simulink subsystem "Pack_SOC_Estimation"  (R2021a)
settings: Solver=VariableStepAuto  StartTime=0.0  StopTime=10.0  RelTol=1e-3
(part 1 of 4)
settings Model: Creator=mirko  LastModifiedBy=mirko

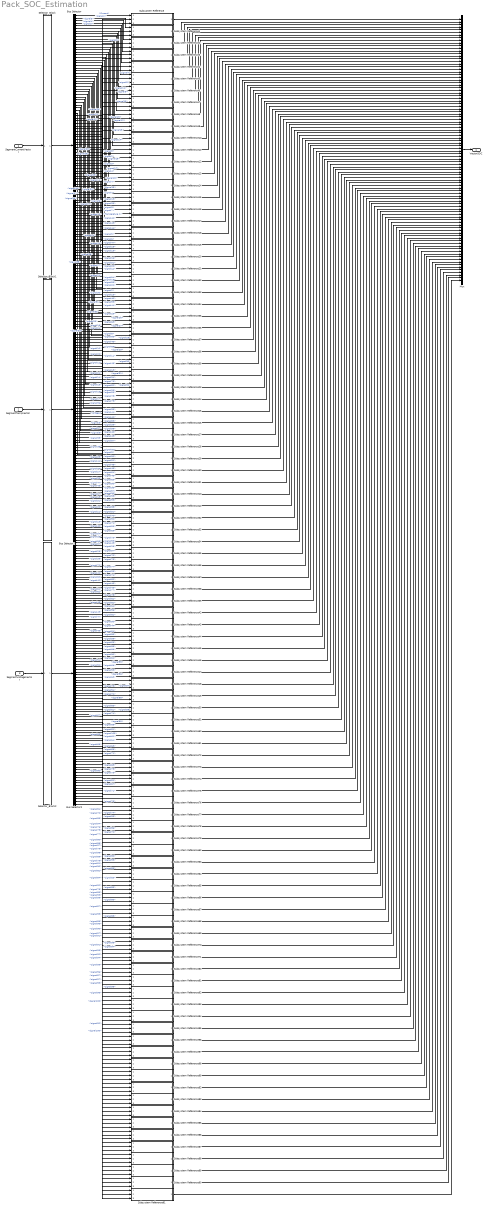
== system Pack_SOC_Estimation ==
  SegmentCurrentVector : Inport
  SegmentTempVector : Inport  Port=2
  SegmentVoltageVector : Inport  Port=3
  Bus Selector : BusSelector  OutputSignals=Current,signal2,signal3,signal4,signal5,signal6,signal7,signal8,signal9,signal10,signal11,signal12,signal13,signal14,signal15,signal16,signal17,signal18,signal19,signal20,signal21,signal22,signal23,signal24,signal25,signal26,signal27,signal28,signal29,signal30,signal31,signal32,signal33,signal34,signal35,signal36,signal37,signal38,signal39,signal40,signal41,signal42,signal43,signal44,signal45,signal46,signal47,signal48,signal49,signal50,signal51,signal52,signal53,signal54,signal55,signal56,signal57,signal58,signal59,signal60,signal61,signal62,signal63,signal64,signal65,signal66,signal67,signal68,signal69,signal70,signal71,signal72,signal73,signal74,signal75,signal76,signal77,signal78,signal79,signal80,signal81,signal82,signal83,signal84,signal85,signal86,signal87,signal88,signal89,signal90,signal91,signal92,signal93,signal94,signal95,signal96,signal97,signal98,signal99,signal100
  Bus Selector1 : BusSelector  OutputSignals=Temperature K,signal2,signal3,signal4,signal5,signal6,signal7,signal8,signal9,signal10,signal11,signal12,signal13,signal14,signal15,signal16,signal17,signal18,signal19,signal20,signal21,signal22,signal23,signal24,signal25,signal26,signal27,signal28,signal29,signal30,signal31,signal32,signal33,signal34,signal35,signal36,signal37,signal38,signal39,signal40,signal41,signal42,signal43,signal44,signal45,signal46,signal47,signal48,signal49,signal50,signal51,signal52,signal53,signal54,signal55,signal56,signal57,signal58,signal59,signal60,signal61,signal62,signal63,signal64,signal65,signal66,signal67,signal68,signal69,signal70,signal71,signal72,signal73,signal74,signal75,signal76,signal77,signal78,signal79,signal80,signal81,signal82,signal83,signal84,signal85,signal86,signal87,signal88,signal89,signal90,signal91,signal92,signal93,signal94,signal95,signal96,signal97,signal98,signal99,signal100
  Bus Selector2 : BusSelector  OutputSignals=Voltage,signal2,signal3,signal4,signal5,signal6,signal7,signal8,signal9,signal10,signal11,signal12,signal13,signal14,signal15,signal16,signal17,signal18,signal19,signal20,signal21,signal22,signal23,signal24,signal25,signal26,signal27,signal28,signal29,signal30,signal31,signal32,signal33,signal34,signal35,signal36,signal37,signal38,signal39,signal40,signal41,signal42,signal43,signal44,signal45,signal46,signal47,signal48,signal49,signal50,signal51,signal52,signal53,signal54,signal55,signal56,signal57,signal58,signal59,signal60,signal61,signal62,signal63,signal64,signal65,signal66,signal67,signal68,signal69,signal70,signal71,signal72,signal73,signal74,signal75,signal76,signal77,signal78,signal79,signal80,signal81,signal82,signal83,signal84,signal85,signal86,signal87,signal88,signal89,signal90,signal91,signal92,signal93,signal94,signal95,signal96,signal97,signal98,signal99,signal100
  Mux : Mux  Inputs=100
  Selector_Block : Subsystem
  Selector_Block1 : Subsystem
  Selector_Block2 : Subsystem
  Subsystem Reference{,1..99} (100 alike) : Subsystem  ReferencedSubsystem=Single_Cell_SOC_Estimation
  VectorSOC : Outport
  wires:
  SegmentCurrentVector/1 -> Selector_Block/1(In1)
  SegmentTempVector/1 -> Selector_Block1/1(In1)
  SegmentVoltageVector/1 -> Selector_Block2/1(In1)
  Bus Selector/1 -> Subsystem Reference/1  "<Current>"
  Bus Selector/2 -> Subsystem Reference1/1  "<signal2>"
  Bus Selector/3 -> Subsystem Reference2/1  "<signal3>"
  Bus Selector/4 -> Subsystem Reference3/1  "<signal4>"
  Bus Selector/5 -> Subsystem Reference4/1  "<signal5>"
  Bus Selector/6 -> Subsystem Reference5/1  "<signal6>"
  Bus Selector/7 -> Subsystem Reference6/1  "<signal7>"
  Bus Selector/8 -> Subsystem Reference7/1  "<signal8>"
  Bus Selector/9 -> Subsystem Reference8/1  "<signal9>"
  Bus Selector/10 -> Subsystem Reference9/1  "<signal10>"
  Bus Selector/11 -> Subsystem Reference10/1  "<signal11>"
  Bus Selector/12 -> Subsystem Reference11/1  "<signal12>"
  Bus Selector/13 -> Subsystem Reference12/1  "<signal13>"
  Bus Selector/14 -> Subsystem Reference13/1  "<signal14>"
  Bus Selector/15 -> Subsystem Reference14/1  "<signal15>"
  Bus Selector/16 -> Subsystem Reference15/1  "<signal16>"
  Bus Selector/17 -> Subsystem Reference16/1  "<signal17>"
  Bus Selector/18 -> Subsystem Reference17/1  "<signal18>"
  Bus Selector/19 -> Subsystem Reference18/1  "<signal19>"
  Bus Selector/20 -> Subsystem Reference19/1  "<signal20>"
  Bus Selector/21 -> Subsystem Reference20/1  "<signal21>"
  Bus Selector/22 -> Subsystem Reference21/1  "<signal22>"
  Bus Selector/23 -> Subsystem Reference32/1  "<signal23>"
  Bus Selector/24 -> Subsystem Reference33/1  "<signal24>"
  Bus Selector/25 -> Subsystem Reference34/1  "<signal25>"
  Bus Selector/26 -> Subsystem Reference35/1  "<signal26>"
  Bus Selector/27 -> Subsystem Reference36/1  "<signal27>"
  Bus Selector/28 -> Subsystem Reference37/1  "<signal28>"
  Bus Selector/29 -> Subsystem Reference38/1  "<signal29>"
  Bus Selector/30 -> Subsystem Reference39/1  "<signal30>"
  Bus Selector/31 -> Subsystem Reference22/1  "<signal31>"
  Bus Selector/32 -> Subsystem Reference23/1  "<signal32>"
  Bus Selector/33 -> Subsystem Reference24/1  "<signal33>"
  Bus Selector/34 -> Subsystem Reference25/1  "<signal34>"
  Bus Selector/35 -> Subsystem Reference26/1  "<signal35>"
  Bus Selector/36 -> Subsystem Reference27/1  "<signal36>"
  Bus Selector/37 -> Subsystem Reference28/1  "<signal37>"
  Bus Selector/38 -> Subsystem Reference29/1  "<signal38>"
  Bus Selector/39 -> Subsystem Reference30/1  "<signal39>"
  Bus Selector/40 -> Subsystem Reference31/1  "<signal40>"
  Bus Selector/41 -> Subsystem Reference40/1  "<signal41>"
  Bus Selector/42 -> Subsystem Reference41/1  "<signal42>"
  Bus Selector/43 -> Subsystem Reference52/1  "<signal43>"
  Bus Selector/44 -> Subsystem Reference53/1  "<signal44>"
  Bus Selector/45 -> Subsystem Reference54/1  "<signal45>"
  Bus Selector/46 -> Subsystem Reference55/1  "<signal46>"
  Bus Selector/47 -> Subsystem Reference56/1  "<signal47>"
  Bus Selector/48 -> Subsystem Reference57/1  "<signal48>"
  Bus Selector/49 -> Subsystem Reference58/1  "<signal49>"
  Bus Selector/50 -> Subsystem Reference59/1  "<signal50>"
  Bus Selector/65 -> Subsystem Reference74/1  "<signal65>"
  Bus Selector/87 -> Subsystem Reference96/1  "<signal87>"
  Bus Selector/97 -> Subsystem Reference88/1  "<signal97>"
  Bus Selector/89 -> Subsystem Reference98/1  "<signal89>"
  Bus Selector/81 -> Subsystem Reference80/1  "<signal81>"
  Bus Selector/90 -> Subsystem Reference99/1  "<signal90>"
  Bus Selector/59 -> Subsystem Reference50/1  "<signal59>"
  Bus Selector/78 -> Subsystem Reference69/1  "<signal78>"
  Bus Selector/86 -> Subsystem Reference95/1  "<signal86>"
  Bus Selector/93 -> Subsystem Reference84/1  "<signal93>"
  Bus Selector/92 -> Subsystem Reference83/1  "<signal92>"
  Bus Selector/52 -> Subsystem Reference43/1  "<signal52>"
  Bus Selector/88 -> Subsystem Reference97/1  "<signal88>"
  Bus Selector/51 -> Subsystem Reference42/1  "<signal51>"
  Bus Selector/54 -> Subsystem Reference45/1  "<signal54>"
  Bus Selector/98 -> Subsystem Reference89/1  "<signal98>"
  Bus Selector/80 -> Subsystem Reference71/1  "<signal80>"
  Bus Selector/84 -> Subsystem Reference93/1  "<signal84>"
  Bus Selector/62 -> Subsystem Reference61/1  "<signal62>"
  Bus Selector/70 -> Subsystem Reference79/1  "<signal70>"
  Bus Selector/83 -> Subsystem Reference92/1  "<signal83>"
  Bus Selector/75 -> Subsystem Reference66/1  "<signal75>"
  Bus Selector/76 -> Subsystem Reference67/1  "<signal76>"
  Bus Selector/68 -> Subsystem Reference77/1  "<signal68>"
  Bus Selector/66 -> Subsystem Reference75/1  "<signal66>"
  Bus Selector/82 -> Subsystem Reference81/1  "<signal82>"
  Bus Selector/69 -> Subsystem Reference78/1  "<signal69>"
  Bus Selector/73 -> Subsystem Reference64/1  "<signal73>"
  Bus Selector/56 -> Subsystem Reference47/1  "<signal56>"
  Bus Selector/96 -> Subsystem Reference87/1  "<signal96>"
  Bus Selector/55 -> Subsystem Reference46/1  "<signal55>"
  Bus Selector/60 -> Subsystem Reference51/1  "<signal60>"
  Bus Selector/95 -> Subsystem Reference86/1  "<signal95>"
  Bus Selector/61 -> Subsystem Reference60/1  "<signal61>"
  Bus Selector/64 -> Subsystem Reference73/1  "<signal64>"
  Bus Selector/99 -> Subsystem Reference90/1  "<signal99>"
  Bus Selector/85 -> Subsystem Reference94/1  "<signal85>"
  Bus Selector/100 -> Subsystem Reference91/1  "<signal100>"
  Bus Selector/79 -> Subsystem Reference70/1  "<signal79>"
  Bus Selector/72 -> Subsystem Reference63/1  "<signal72>"
  Bus Selector/77 -> Subsystem Reference68/1  "<signal77>"
  Bus Selector/63 -> Subsystem Reference72/1  "<signal63>"
  Bus Selector/74 -> Subsystem Reference65/1  "<signal74>"
  Bus Selector/57 -> Subsystem Reference48/1  "<signal57>"
  Bus Selector/71 -> Subsystem Reference62/1  "<signal71>"
  Bus Selector/53 -> Subsystem Reference44/1  "<signal53>"
  Bus Selector/58 -> Subsystem Reference49/1  "<signal58>"
  Bus Selector/94 -> Subsystem Reference85/1  "<signal94>"
  Bus Selector/67 -> Subsystem Reference76/1  "<signal67>"
  Bus Selector/91 -> Subsystem Reference82/1  "<signal91>"
  Bus Selector1/79 -> Subsystem Reference70/2  "<signal79>"
  Bus Selector1/69 -> Subsystem Reference78/2  "<signal69>"
  Bus Selector1/67 -> Subsystem Reference76/2  "<signal67>"
  Bus Selector1/66 -> Subsystem Reference75/2  "<signal66>"
  Bus Selector1/46 -> Subsystem Reference55/2  "<signal46>"
  Bus Selector1/70 -> Subsystem Reference79/2  "<signal70>"
  Bus Selector1/24 -> Subsystem Reference33/2  "<signal24>"
  Bus Selector1/29 -> Subsystem Reference38/2  "<signal29>"
  Bus Selector1/37 -> Subsystem Reference28/2  "<signal37>"
  Bus Selector1/47 -> Subsystem Reference56/2  "<signal47>"
  Bus Selector1/39 -> Subsystem Reference30/2  "<signal39>"
  Bus Selector1/31 -> Subsystem Reference22/2  "<signal31>"
  Bus Selector1/40 -> Subsystem Reference31/2  "<signal40>"
  Bus Selector1/27 -> Subsystem Reference36/2  "<signal27>"
  Bus Selector1/23 -> Subsystem Reference32/2  "<signal23>"
  Bus Selector1/9 -> Subsystem Reference8/2  "<signal9>"
  Bus Selector1/75 -> Subsystem Reference66/2  "<signal75>"
  Bus Selector1/78 -> Subsystem Reference69/2  "<signal78>"
  Bus Selector1/77 -> Subsystem Reference68/2  "<signal77>"
  Bus Selector1/25 -> Subsystem Reference34/2  "<signal25>"
  Bus Selector1/76 -> Subsystem Reference67/2  "<signal76>"
  Bus Selector1/61 -> Subsystem Reference60/2  "<signal61>"
  Bus Selector1/62 -> Subsystem Reference61/2  "<signal62>"
  Bus Selector1/65 -> Subsystem Reference74/2  "<signal65>"
  Bus Selector1/63 -> Subsystem Reference72/2  "<signal63>"
  Bus Selector1/80 -> Subsystem Reference71/2  "<signal80>"
  Bus Selector1/53 -> Subsystem Reference44/2  "<signal53>"
  Bus Selector1/52 -> Subsystem Reference43/2  "<signal52>"
  Bus Selector1/51 -> Subsystem Reference42/2  "<signal51>"
  Bus Selector1/54 -> Subsystem Reference45/2  "<signal54>"
  Bus Selector1/93 -> Subsystem Reference84/2  "<signal93>"
  Bus Selector1/94 -> Subsystem Reference85/2  "<signal94>"
  Bus Selector1/91 -> Subsystem Reference82/2  "<signal91>"
  Bus Selector1/82 -> Subsystem Reference81/2  "<signal82>"
  Bus Selector1/81 -> Subsystem Reference80/2  "<signal81>"
  Bus Selector1/28 -> Subsystem Reference37/2  "<signal28>"
  Bus Selector1/57 -> Subsystem Reference48/2  "<signal57>"
  Bus Selector1/72 -> Subsystem Reference63/2  "<signal72>"
  Bus Selector1/96 -> Subsystem Reference87/2  "<signal96>"
  Bus Selector1/36 -> Subsystem Reference27/2  "<signal36>"
  Bus Selector1/90 -> Subsystem Reference99/2  "<signal90>"
  Bus Selector1/83 -> Subsystem Reference92/2  "<signal83>"
  Bus Selector1/71 -> Subsystem Reference62/2  "<signal71>"
  Bus Selector1/15 -> Subsystem Reference14/2  "<signal15>"
  Bus Selector1/100 -> Subsystem Reference91/2  "<signal100>"
  Bus Selector1/73 -> Subsystem Reference64/2  "<signal73>"
  Bus Selector1/99 -> Subsystem Reference90/2  "<signal99>"
  Bus Selector1/98 -> Subsystem Reference89/2  "<signal98>"
  Bus Selector1/43 -> Subsystem Reference52/2  "<signal43>"
  Bus Selector1/56 -> Subsystem Reference47/2  "<signal56>"
  Bus Selector1/42 -> Subsystem Reference41/2  "<signal42>"
  Bus Selector1/2 -> Subsystem Reference1/2  "<signal2>"
  Bus Selector1/38 -> Subsystem Reference29/2  "<signal38>"
  Bus Selector1/95 -> Subsystem Reference86/2  "<signal95>"
  Bus Selector1/59 -> Subsystem Reference50/2  "<signal59>"
  Bus Selector1/1 -> Subsystem Reference/2  "<Temperature K>"
  Bus Selector1/58 -> Subsystem Reference49/2  "<signal58>"
  Bus Selector1/4 -> Subsystem Reference3/2  "<signal4>"
  Bus Selector1/88 -> Subsystem Reference97/2  "<signal88>"
  Bus Selector1/48 -> Subsystem Reference57/2  "<signal48>"
  Bus Selector1/30 -> Subsystem Reference39/2  "<signal30>"
  Bus Selector1/34 -> Subsystem Reference25/2  "<signal34>"
  Bus Selector1/84 -> Subsystem Reference93/2  "<signal84>"
  Bus Selector1/86 -> Subsystem Reference95/2  "<signal86>"
  Bus Selector1/12 -> Subsystem Reference11/2  "<signal12>"
  Bus Selector1/20 -> Subsystem Reference19/2  "<signal20>"
  Bus Selector1/33 -> Subsystem Reference24/2  "<signal33>"
  Bus Selector1/26 -> Subsystem Reference35/2  "<signal26>"
  Bus Selector1/89 -> Subsystem Reference98/2  "<signal89>"
  Bus Selector1/18 -> Subsystem Reference17/2  "<signal18>"
  Bus Selector1/16 -> Subsystem Reference15/2  "<signal16>"
  Bus Selector1/85 -> Subsystem Reference94/2  "<signal85>"
  Bus Selector1/74 -> Subsystem Reference65/2  "<signal74>"
  Bus Selector1/32 -> Subsystem Reference23/2  "<signal32>"
  Bus Selector1/68 -> Subsystem Reference77/2  "<signal68>"
  Bus Selector1/97 -> Subsystem Reference88/2  "<signal97>"
  Bus Selector1/19 -> Subsystem Reference18/2  "<signal19>"
  Bus Selector1/6 -> Subsystem Reference5/2  "<signal6>"
  Bus Selector1/5 -> Subsystem Reference4/2  "<signal5>"
  Bus Selector1/10 -> Subsystem Reference9/2  "<signal10>"
  Bus Selector1/45 -> Subsystem Reference54/2  "<signal45>"
  Bus Selector1/11 -> Subsystem Reference10/2  "<signal11>"
  Bus Selector1/14 -> Subsystem Reference13/2  "<signal14>"
  Bus Selector1/49 -> Subsystem Reference58/2  "<signal49>"
  Bus Selector1/60 -> Subsystem Reference51/2  "<signal60>"
  Bus Selector1/35 -> Subsystem Reference26/2  "<signal35>"
  Bus Selector1/64 -> Subsystem Reference73/2  "<signal64>"
  Bus Selector1/50 -> Subsystem Reference59/2  "<signal50>"
  Bus Selector1/22 -> Subsystem Reference21/2  "<signal22>"
  Bus Selector1/13 -> Subsystem Reference12/2  "<signal13>"
  Bus Selector1/7 -> Subsystem Reference6/2  "<signal7>"
  Bus Selector1/21 -> Subsystem Reference20/2  "<signal21>"
  Bus Selector1/3 -> Subsystem Reference2/2  "<signal3>"
  Bus Selector1/8 -> Subsystem Reference7/2  "<signal8>"
  Bus Selector1/55 -> Subsystem Reference46/2  "<signal55>"
  Bus Selector1/44 -> Subsystem Reference53/2  "<signal44>"
  Bus Selector1/92 -> Subsystem Reference83/2  "<signal92>"
  Bus Selector1/17 -> Subsystem Reference16/2  "<signal17>"
  Bus Selector1/41 -> Subsystem Reference40/2  "<signal41>"
  Bus Selector1/87 -> Subsystem Reference96/2  "<signal87>"
  Bus Selector2/79 -> Subsystem Reference70/3  "<signal79>"
  Bus Selector2/69 -> Subsystem Reference78/3  "<signal69>"
  Bus Selector2/67 -> Subsystem Reference76/3  "<signal67>"
  Bus Selector2/66 -> Subsystem Reference75/3  "<signal66>"
  Bus Selector2/46 -> Subsystem Reference55/3  "<signal46>"
  Bus Selector2/70 -> Subsystem Reference79/3  "<signal70>"
  Bus Selector2/24 -> Subsystem Reference33/3  "<signal24>"
  Bus Selector2/29 -> Subsystem Reference38/3  "<signal29>"
  Bus Selector2/37 -> Subsystem Reference28/3  "<signal37>"
  Bus Selector2/47 -> Subsystem Reference56/3  "<signal47>"
  Bus Selector2/39 -> Subsystem Reference30/3  "<signal39>"
  Bus Selector2/31 -> Subsystem Reference22/3  "<signal31>"
  Bus Selector2/40 -> Subsystem Reference31/3  "<signal40>"
  Bus Selector2/27 -> Subsystem Reference36/3  "<signal27>"
  Bus Selector2/23 -> Subsystem Reference32/3  "<signal23>"
  Bus Selector2/9 -> Subsystem Reference8/3  "<signal9>"
  Bus Selector2/75 -> Subsystem Reference66/3  "<signal75>"
  Bus Selector2/78 -> Subsystem Reference69/3  "<signal78>"
  Bus Selector2/77 -> Subsystem Reference68/3  "<signal77>"
  Bus Selector2/25 -> Subsystem Reference34/3  "<signal25>"
  Bus Selector2/76 -> Subsystem Reference67/3  "<signal76>"
  Bus Selector2/61 -> Subsystem Reference60/3  "<signal61>"
  Bus Selector2/62 -> Subsystem Reference61/3  "<signal62>"
  Bus Selector2/65 -> Subsystem Reference74/3  "<signal65>"
  Bus Selector2/63 -> Subsystem Reference72/3  "<signal63>"
  Bus Selector2/80 -> Subsystem Reference71/3  "<signal80>"
  Bus Selector2/53 -> Subsystem Reference44/3  "<signal53>"
  Bus Selector2/52 -> Subsystem Reference43/3  "<signal52>"
  Bus Selector2/51 -> Subsystem Reference42/3  "<signal51>"
  Bus Selector2/54 -> Subsystem Reference45/3  "<signal54>"
  Bus Selector2/93 -> Subsystem Reference84/3  "<signal93>"
  Bus Selector2/94 -> Subsystem Reference85/3  "<signal94>"
  Bus Selector2/91 -> Subsystem Reference82/3  "<signal91>"
  Bus Selector2/82 -> Subsystem Reference81/3  "<signal82>"
  Bus Selector2/81 -> Subsystem Reference80/3  "<signal81>"
  Bus Selector2/28 -> Subsystem Reference37/3  "<signal28>"
  Bus Selector2/57 -> Subsystem Reference48/3  "<signal57>"
  Bus Selector2/72 -> Subsystem Reference63/3  "<signal72>"
  Bus Selector2/96 -> Subsystem Reference87/3  "<signal96>"
  Bus Selector2/36 -> Subsystem Reference27/3  "<signal36>"
  Bus Selector2/90 -> Subsystem Reference99/3  "<signal90>"
  Bus Selector2/83 -> Subsystem Reference92/3  "<signal83>"
  Bus Selector2/71 -> Subsystem Reference62/3  "<signal71>"
  Bus Selector2/15 -> Subsystem Reference14/3  "<signal15>"
  Bus Selector2/100 -> Subsystem Reference91/3  "<signal100>"
  Bus Selector2/73 -> Subsystem Reference64/3  "<signal73>"
  Bus Selector2/99 -> Subsystem Reference90/3  "<signal99>"
  Bus Selector2/98 -> Subsystem Reference89/3  "<signal98>"
  Bus Selector2/43 -> Subsystem Reference52/3  "<signal43>"
  Bus Selector2/56 -> Subsystem Reference47/3  "<signal56>"
  Bus Selector2/42 -> Subsystem Reference41/3  "<signal42>"
  Bus Selector2/2 -> Subsystem Reference1/3  "<signal2>"
  Bus Selector2/38 -> Subsystem Reference29/3  "<signal38>"
  Bus Selector2/95 -> Subsystem Reference86/3  "<signal95>"
  Bus Selector2/59 -> Subsystem Reference50/3  "<signal59>"
  Bus Selector2/1 -> Subsystem Reference/3  "<Voltage>"
  Bus Selector2/58 -> Subsystem Reference49/3  "<signal58>"
  Bus Selector2/4 -> Subsystem Reference3/3  "<signal4>"
  Bus Selector2/88 -> Subsystem Reference97/3  "<signal88>"
  Bus Selector2/48 -> Subsystem Reference57/3  "<signal48>"
  Bus Selector2/30 -> Subsystem Reference39/3  "<signal30>"
  Bus Selector2/34 -> Subsystem Reference25/3  "<signal34>"
  Bus Selector2/84 -> Subsystem Reference93/3  "<signal84>"
  Bus Selector2/86 -> Subsystem Reference95/3  "<signal86>"
  Bus Selector2/12 -> Subsystem Reference11/3  "<signal12>"
  Bus Selector2/20 -> Subsystem Reference19/3  "<signal20>"
  Bus Selector2/33 -> Subsystem Reference24/3  "<signal33>"
  Bus Selector2/26 -> Subsystem Reference35/3  "<signal26>"
  Bus Selector2/89 -> Subsystem Reference98/3  "<signal89>"
  Bus Selector2/18 -> Subsystem Reference17/3  "<signal18>"
  Bus Selector2/16 -> Subsystem Reference15/3  "<signal16>"
  Bus Selector2/85 -> Subsystem Reference94/3  "<signal85>"
  Bus Selector2/74 -> Subsystem Reference65/3  "<signal74>"
  Bus Selector2/32 -> Subsystem Reference23/3  "<signal32>"
  Bus Selector2/68 -> Subsystem Reference77/3  "<signal68>"
  Bus Selector2/97 -> Subsystem Reference88/3  "<signal97>"
  Bus Selector2/19 -> Subsystem Reference18/3  "<signal19>"
  Bus Selector2/6 -> Subsystem Reference5/3  "<signal6>"
  Bus Selector2/5 -> Subsystem Reference4/3  "<signal5>"
  Bus Selector2/10 -> Subsystem Reference9/3  "<signal10>"
  Bus Selector2/45 -> Subsystem Reference54/3  "<signal45>"
  Bus Selector2/11 -> Subsystem Reference10/3  "<signal11>"
  Bus Selector2/14 -> Subsystem Reference13/3  "<signal14>"
  Bus Selector2/49 -> Subsystem Reference58/3  "<signal49>"
  Bus Selector2/60 -> Subsystem Reference51/3  "<signal60>"
  Bus Selector2/35 -> Subsystem Reference26/3  "<signal35>"
  Bus Selector2/64 -> Subsystem Reference73/3  "<signal64>"
  Bus Selector2/50 -> Subsystem Reference59/3  "<signal50>"
  Bus Selector2/22 -> Subsystem Reference21/3  "<signal22>"
  Bus Selector2/13 -> Subsystem Reference12/3  "<signal13>"
  Bus Selector2/7 -> Subsystem Reference6/3  "<signal7>"
  Bus Selector2/21 -> Subsystem Reference20/3  "<signal21>"
  Bus Selector2/3 -> Subsystem Reference2/3  "<signal3>"
  Bus Selector2/8 -> Subsystem Reference7/3  "<signal8>"
  Bus Selector2/55 -> Subsystem Reference46/3  "<signal55>"
  Bus Selector2/44 -> Subsystem Reference53/3  "<signal44>"
  Bus Selector2/92 -> Subsystem Reference83/3  "<signal92>"
  Bus Selector2/17 -> Subsystem Reference16/3  "<signal17>"
  Bus Selector2/41 -> Subsystem Reference40/3  "<signal41>"
  Bus Selector2/87 -> Subsystem Reference96/3  "<signal87>"
  Mux/1 -> VectorSOC/1
  Subsystem Reference/1 -> Mux/1
  Subsystem Reference1/1 -> Mux/2
  Subsystem Reference2/1 -> Mux/3
  Subsystem Reference3/1 -> Mux/4
  Subsystem Reference4/1 -> Mux/5
  Subsystem Reference5/1 -> Mux/6
  Subsystem Reference6/1 -> Mux/7
  Subsystem Reference7/1 -> Mux/8
  Subsystem Reference8/1 -> Mux/9
  Subsystem Reference9/1 -> Mux/10
  Subsystem Reference10/1 -> Mux/11
  Subsystem Reference11/1 -> Mux/12
  Subsystem Reference12/1 -> Mux/13
  Subsystem Reference15/1 -> Mux/16
  Subsystem Reference13/1 -> Mux/14
  Subsystem Reference16/1 -> Mux/17
  Subsystem Reference32/1 -> Mux/23
  Subsystem Reference34/1 -> Mux/25
  Subsystem Reference21/1 -> Mux/22
  Subsystem Reference14/1 -> Mux/15
  Subsystem Reference19/1 -> Mux/20
  Subsystem Reference35/1 -> Mux/26
  Subsystem Reference18/1 -> Mux/19
  Subsystem Reference33/1 -> Mux/24
  Subsystem Reference17/1 -> Mux/18
  Subsystem Reference20/1 -> Mux/21
  Subsystem Reference38/1 -> Mux/29
  Subsystem Reference52/1 -> Mux/43
  Subsystem Reference55/1 -> Mux/46
  Subsystem Reference58/1 -> Mux/49
  Subsystem Reference36/1 -> Mux/27
  Subsystem Reference39/1 -> Mux/30
  Subsystem Reference27/1 -> Mux/36
  Subsystem Reference53/1 -> Mux/44
  Subsystem Reference57/1 -> Mux/48
  Subsystem Reference31/1 -> Mux/40
  Subsystem Reference41/1 -> Mux/42
  Subsystem Reference29/1 -> Mux/38
  Subsystem Reference40/1 -> Mux/41
  Subsystem Reference23/1 -> Mux/32
  Subsystem Reference42/1 -> Mux/51
  Subsystem Reference56/1 -> Mux/47
  Subsystem Reference54/1 -> Mux/45
  Subsystem Reference26/1 -> Mux/35
  Subsystem Reference37/1 -> Mux/28
  Subsystem Reference24/1 -> Mux/33
  Subsystem Reference30/1 -> Mux/39
  Subsystem Reference43/1 -> Mux/52
  Subsystem Reference28/1 -> Mux/37
  Subsystem Reference22/1 -> Mux/31
  Subsystem Reference59/1 -> Mux/50
  Subsystem Reference25/1 -> Mux/34
  Selector_Block/1(OutBus) -> Bus Selector/1
  Selector_Block1/1(OutBus) -> Bus Selector1/1
  Selector_Block2/1(OutBus) -> Bus Selector2/1
  Subsystem Reference47/1 -> Mux/56
  Subsystem Reference44/1 -> Mux/53
  Subsystem Reference50/1 -> Mux/59
  Subsystem Reference46/1 -> Mux/55
  Subsystem Reference49/1 -> Mux/58
  Subsystem Reference45/1 -> Mux/54
  Subsystem Reference48/1 -> Mux/57
  Subsystem Reference61/1 -> Mux/62
  Subsystem Reference67/1 -> Mux/76
  Subsystem Reference70/1 -> Mux/79
  Subsystem Reference81/1 -> Mux/82
  Subsystem Reference51/1 -> Mux/60
  Subsystem Reference72/1 -> Mux/63
  Subsystem Reference78/1 -> Mux/69
  Subsystem Reference68/1 -> Mux/77
  Subsystem Reference80/1 -> Mux/81
  Subsystem Reference64/1 -> Mux/73
  Subsystem Reference66/1 -> Mux/75
  Subsystem Reference62/1 -> Mux/71
  Subsystem Reference65/1 -> Mux/74
  Subsystem Reference74/1 -> Mux/65
  Subsystem Reference93/1 -> Mux/84
  Subsystem Reference71/1 -> Mux/80
  Subsystem Reference69/1 -> Mux/78
  Subsystem Reference77/1 -> Mux/68
  Subsystem Reference60/1 -> Mux/61
  Subsystem Reference75/1 -> Mux/66
  Subsystem Reference63/1 -> Mux/72
  Subsystem Reference94/1 -> Mux/85
  Subsystem Reference79/1 -> Mux/70
  Subsystem Reference73/1 -> Mux/64
  Subsystem Reference92/1 -> Mux/83
  Subsystem Reference76/1 -> Mux/67
  Subsystem Reference97/1 -> Mux/88
  Subsystem Reference95/1 -> Mux/86
  Subsystem Reference98/1 -> Mux/89
  Subsystem Reference86/1 -> Mux/95
  Subsystem Reference90/1 -> Mux/99
  Subsystem Reference88/1 -> Mux/97
  Subsystem Reference85/1 -> Mux/94
  Subsystem Reference96/1 -> Mux/87
  Subsystem Reference83/1 -> Mux/92
  Subsystem Reference89/1 -> Mux/98
  Subsystem Reference82/1 -> Mux/91
  Subsystem Reference87/1 -> Mux/96
  Subsystem Reference99/1 -> Mux/90
  Subsystem Reference84/1 -> Mux/93
  Subsystem Reference91/1 -> Mux/100
